simulink model "multiportselector_tut1"  (Simulink 5.0)
settings: Solver=FixedStepDiscrete  StartTime=0.0  StopTime=10.0  RelTol=1e-3
PreLoadFcn:
  | dsp_examples_A = [1:10;1 1 0 0 1 1 0 0 1 1]';
PostLoadFcn:
  | set_param(gcs,'SimulationCommand','Update')
libraries: dspindex x1, dspsrcs4 x1
settings Model: RequirementInfo=9  Creator=ckamachi  LastModifiedBy=cclarke  ExtModeTrigMode=oneshot  ExtModeArmWhenConnect=off  LimitDataPoints=off  SignalLoggingName=logsOut  BlockReductionOpt=off  BooleanDataType=off  ZeroCrossControl=UseLocalSettings  RTWMathFcnLibMatFile=iso_c_tmw.mat

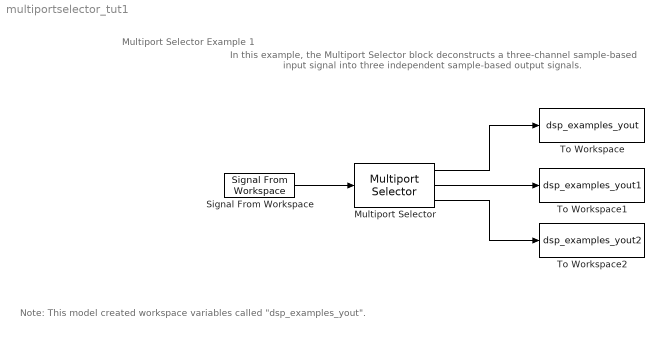
== system multiportselector_tut1 ==
  note: Multiport Selector Example 1
  note: In this example, the Multiport Selector block deconstructs
      | a three-channel sample-based input signal into three
      | independent sample-based output signals.
  note: Note: This model created workspace variables called "dsp_examples_yout".
  Multiport Selector : dspindex/Multiport Selector  rowsOrCols=Rows  idxCellArray={ 1, 2, 3 }  idxErrMode=Clip Index
  Signal From Workspace : dspsrcs4/Signal From Workspace  X=randn(3,1,10)  Ts=1  nsamps=1  OutputAfterFinalValue=Setting to zero
  To Workspace : ToWorkspace  VariableName=dsp_examples_yout  SampleTime=-1  SaveFormat=Array
  To Workspace1 : ToWorkspace  VariableName=dsp_examples_yout1  SampleTime=-1  SaveFormat=Array
  To Workspace2 : ToWorkspace  VariableName=dsp_examples_yout2  SampleTime=-1  SaveFormat=Array
  wires:
  Signal From Workspace/1 -> Multiport Selector/1
  Multiport Selector/1 -> To Workspace/1
  Multiport Selector/3 -> To Workspace2/1
  Multiport Selector/2 -> To Workspace1/1
